simulink model "modelIntegrator"  (R2015a)
settings: Solver=ode45  StartTime=0.0  StopTime=10.0  RelTol=1e-3
values from neighbouring files (symbols this model uses):
  A = [-R/L,0,0 ... (first row only)    [script.m]    (also in scriptadaptive.m)
  B = [1/L; 0; 0]    [script.m]    (also in scriptadaptive.m)
  Cy = [ 0,1,0]    [script.m]    (also in scriptadaptive.m)
  D = 0    [script.m]    (also in scriptadaptive.m = [0])
  denC = [M C K]    [script.m]    (also in scriptadaptive.m)
  denM = [L R]    [script.m]    (also in scriptadaptive.m)
  klqi = lqi(sys, 0.1*eye(4),1,zeros(4,1))    [script.m]
  numC = Gamma    (= -206.8)    [script.m]    (also in scriptadaptive.m)
undefined symbols (not defined in the file or in its folder): Continuous, Time
libraries: ctrlSharedLib x1
settings Model: Creator=user  LastModifiedBy=user

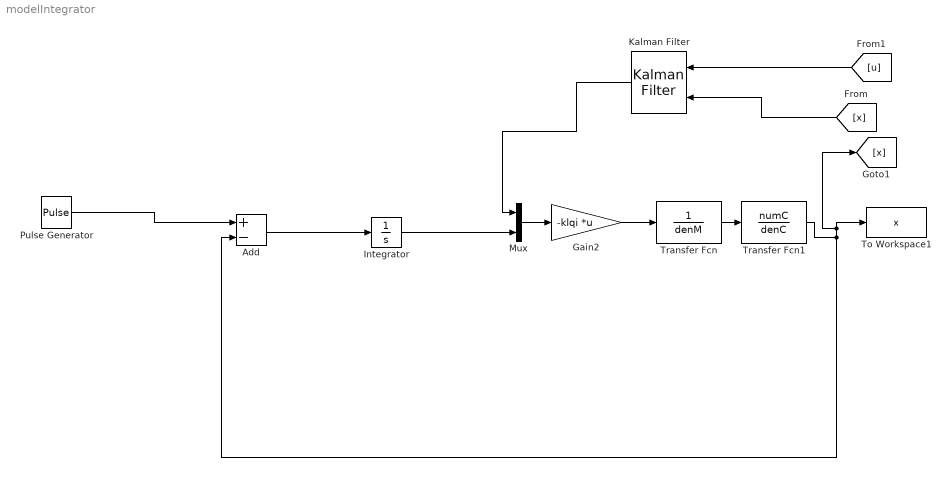
== system modelIntegrator ==
  Add : Sum  Inputs=+-
  Gain2 : Gain  Gain=-klqi  Multiplication=Matrix(K*u)
  Integrator : Integrator
  Kalman Filter : ctrlSharedLib/Kalman Filter  TimeDomain=Continuous-Time  UseCurrentEstimator=on  ModelSource=Individual A, B, C, D matrices  ModelSourceVariable=ss(0.95,1,1,0,1)  A=A  B=B  C=Cy  D=D  NumberOfStates=1  NumberOfInputs=1  NumberOfOutputs=1  InitialEstimateSource=Dialog  X0=0  P0=10  UseK=off  UseGH=off  NumberOfProcessNoiseInputs=1  G=1  TimeInvariantG=on  H=0  TimeInvariantH=on  Q=0.000001  TimeInvariantQ=on  R=0.000001  TimeInvariantR=on  N=0  TimeInvariantN=on  AddInputPort=on  AddEnablePort=off  ExternalReset=none  OutputEstimatedY=off  OutputP=off  Ts=1/200
  Mux : Mux  Inputs=2
  Pulse Generator : DiscretePulseGenerator  PulseType=Time based  Period=10  PulseWidth=50  PhaseDelay=5
  To Workspace1 : ToWorkspace  VariableName=x  SaveFormat=Timeseries  SampleTime=1/200
  Transfer Fcn : TransferFcn  Denominator=denM
  Transfer Fcn1 : TransferFcn  Numerator=numC  Denominator=denC
  wires:
  Transfer Fcn/1 -> Transfer Fcn1/1
  Transfer Fcn1/1 -> [x], To Workspace1/1, Add/2
  [x] -> Kalman Filter/2
  [u] -> Kalman Filter/1
  Pulse Generator/1 -> Add/1
  Gain2/1 -> Transfer Fcn/1
  Mux/1 -> Gain2/1
  Add/1 -> Integrator/1
  Integrator/1 -> Mux/2
  Kalman Filter/1 -> Mux/1
